simulink model "Copy_of_pll05"  (Simulink 8.1)
settings: Solver=ode45  StartTime=0.0  StopTime=100  MaxStep=0.0001  RelTol=1e-3
values from neighbouring files (symbols this model uses):
  delay_t1 = delay_t(i)    [nw_pll01.m]    (also in pll4.m = 0.2; pll5.m)
  delay_t2 = delay_t(i+1)    [nw_pll01.m]    (also in pll4.m = 0.16; pll5.m)
  delay_t3 = delay_t(i+2)    [nw_pll01.m]    (also in pll4.m = 0.13; pll5.m)
libraries: commsynccomp2 x1, simulink x1
settings Model: Creator=my88899  LastModifiedBy=my88899
settings DataIOCC: SignalLoggingSaveFormat=Dataset
settings OptimizationCC: ExpressionDepthLimit=128
settings DebuggingCC: FcnCallInpInsideContextMsg=EnableAllAsError
settings GRTTargetCC: CombineOutputUpdateFcns=on  GRTInterface=off

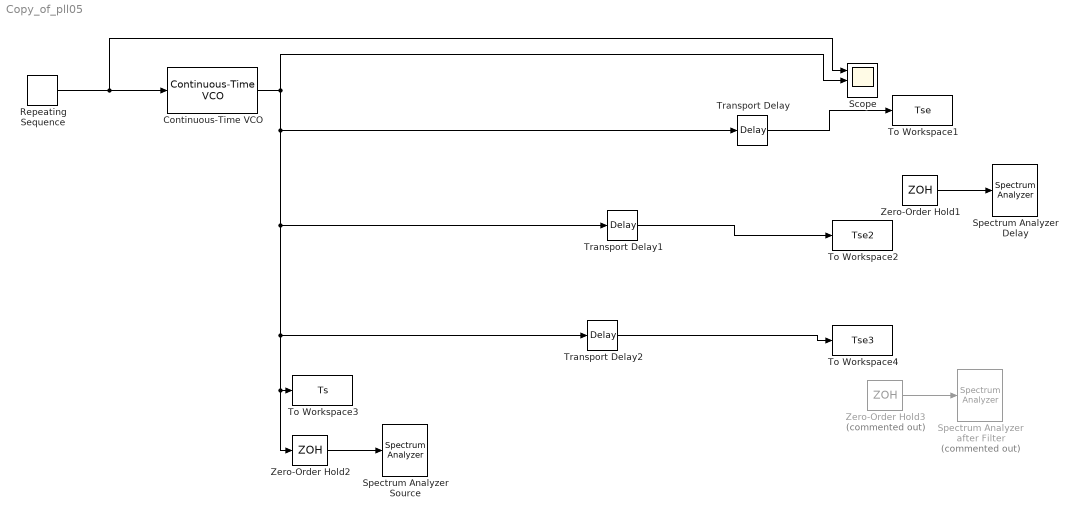
== system Copy_of_pll05 ==
  Continuous-Time VCO : commsynccomp2/Continuous-Time VCO  Ac=5  Fc=100  Kc=100  Ph=0
  Repeating Sequence : simulink/Sources/Repeating Sequence  rep_seq_t=[0 1]  rep_seq_y=[0 5]
  Scope : Scope  NumInputPorts=3
      settings: TimeRange=0.1038961038961048  YMin=5.645~-5~-5  YMax=5.7~5~5  MaxDataPoints=100000
  "Spectrum Analyzer Delay " : SpectrumAnalyzer
      settings: CopyFcn=scopeextensions.ScopeBlock.callback(gcbh, 'onBlockCopy', gcbh);  DeleteFcn=scopeextensions.ScopeBlock.callback(gcbh, 'onBlockDelete');  PreSaveFcn=scopeextensions.ScopeBlock.callback(gcbh, 'onModelSave');  NameChangeFcn=scopeextensions.ScopeBlock.callback(gcbh, 'onBlockRename');  CloseFcn=scopeextensions.ScopeBlock.callback(gcbh, 'onBlockClose');  PreDeleteFcn=scopeextensions.ScopeBlock.callback(gcbh, 'onBlockPreDelete');
  "Spectrum Analyzer Source " : SpectrumAnalyzer
      settings: CopyFcn=scopeextensions.ScopeBlock.callback(gcbh, 'onBlockCopy', gcbh);  DeleteFcn=scopeextensions.ScopeBlock.callback(gcbh, 'onBlockDelete');  PreSaveFcn=scopeextensions.ScopeBlock.callback(gcbh, 'onModelSave');  NameChangeFcn=scopeextensions.ScopeBlock.callback(gcbh, 'onBlockRename');  CloseFcn=scopeextensions.ScopeBlock.callback(gcbh, 'onBlockClose');  PreDeleteFcn=scopeextensions.ScopeBlock.callback(gcbh, 'onBlockPreDelete');
  "Spectrum Analyzer after Filter " : SpectrumAnalyzer  Commented=on
      settings: CopyFcn=scopeextensions.ScopeBlock.callback(gcbh, 'onBlockCopy', gcbh);  DeleteFcn=scopeextensions.ScopeBlock.callback(gcbh, 'onBlockDelete');  PreSaveFcn=scopeextensions.ScopeBlock.callback(gcbh, 'onModelSave');  NameChangeFcn=scopeextensions.ScopeBlock.callback(gcbh, 'onBlockRename');  CloseFcn=scopeextensions.ScopeBlock.callback(gcbh, 'onBlockClose');  PreDeleteFcn=scopeextensions.ScopeBlock.callback(gcbh, 'onBlockPreDelete');
  To Workspace1 : ToWorkspace  VariableName=Tse  SampleTime=-1  SaveFormat=Timeseries
  To Workspace2 : ToWorkspace  VariableName=Tse2  SampleTime=-1  SaveFormat=Timeseries
  To Workspace3 : ToWorkspace  VariableName=Ts  SampleTime=-1  SaveFormat=Timeseries
  To Workspace4 : ToWorkspace  VariableName=Tse3  SampleTime=-1  SaveFormat=Timeseries
  Transport Delay : TransportDelay  DelayTime=delay_t1
  Transport Delay1 : TransportDelay  DelayTime=delay_t2
  Transport Delay2 : TransportDelay  DelayTime=delay_t3
  Zero-Order Hold1 : ZeroOrderHold  SampleTime=0.01
  Zero-Order Hold2 : ZeroOrderHold  SampleTime=0.01
  Zero-Order Hold3 : ZeroOrderHold  Commented=on  SampleTime=0.01
  wires:
  Repeating Sequence/1 -> Scope/1, Continuous-Time VCO/1
  Zero-Order Hold1/1 -> "Spectrum Analyzer Delay "/1
  Zero-Order Hold2/1 -> "Spectrum Analyzer Source "/1
  Continuous-Time VCO/1 -> Transport Delay/1, Transport Delay1/1, Transport Delay2/1, Zero-Order Hold2/1, To Workspace3/1, Scope/2
  Zero-Order Hold3/1 -> "Spectrum Analyzer after Filter "/1
  Transport Delay/1 -> To Workspace1/1
  Transport Delay1/1 -> To Workspace2/1
  Transport Delay2/1 -> To Workspace4/1
